simulink model "SensorFaultInj"  (R2013a)
settings: Solver=FixedStepDiscrete  SolverMode=SingleTasking  StartTime=0.0  StopTime=SimLength  FixedStep=SampleTime  RelTol=1e-3
values from neighbouring files (symbols this model uses):
  GlobalSeed = 10    [start_framework07.m]
  SampleTime = 0.01    [start_framework07.m]
  SimLength = 40    [start_framework07.m]
undefined symbols (not defined in the file or in its folder): DiscIntNeverNeededParam
libraries: dspswit3 x48, simulink x32
(part 5 of 9)

== system SensorFaultInj/FIM_Muster1/Parser Modul/schedule once per sample step /schedule_fcn id 2 ==
  In1 : Inport
  Discrete-Time Integrator : DiscreteIntegrator  SampleTime=-1  ICPrevOutput=DiscIntNeverNeededParam  ICPrevScaledInput=DiscIntNeverNeededParam
  Scope1 : Scope  NumInputPorts=2
      settings: YMin=-5~-5  YMax=5~5  SaveName=ScopeData25
  SimLength : Constant  Value=SimLength
  ex_sfun_schedulefcn1 : S-Function  FunctionName=ex_sfun_schedulefcn  EnableBusSupport=off  mask(Legacy Function){SFunctionSpec=single y1 = schedule_fcn(double u1, double u2, single u3, single u4), ShowSpec=on}
      mask prompts: ShowSpec "Display function specification"
      mask help:
      | This block allows you to call the legacy functions specified by the following Legacy Code Tool definition:
      | def.SFunctionName = 'ex_sfun_schedulefcn';
      | def.OutputFcnSpec = 'single y1 = schedule_fcn(double u1, double u2, single u3, single u4)';
      | def.HeaderFiles = {'schedule_fcn.hpp'};
      | def.SourceFiles = {'schedule_fcn.cpp'};
      | def.Options.language = 'C++';
      mask Help: <p>This block was generated automatically by the Legacy Code Tool. For detailed help on this tool, call<a href="matlab:legacy_code('help')"> legacy_code('help')</a>.</p>
      mask Callback ShowSpec:
      | if strcmp(get_param(gcbh, 'ShowSpec'), 'on')
      |   set_param(gcbh, 'MaskDisplay', sprintf('fprintf(''%s'');', get_param(gcbh, 'SFunctionSpec')));
      | else
      |   set_param(gcbh, 'MaskDisplay', sprintf('fprintf(''%s'');', get_param(gcbh, 'FunctionName')));
      | end
      mask Display: fprintf('single y1 = schedule_fcn(double u1, double u2, single u3, single u4)');
  "fault_id " : Constant  Value=2  OutDataTypeStr=single
  one : Constant
  output : Outport  OutputWhenDisabled=reset  InitialOutput=[0]
  wires:
  one/1 -> Discrete-Time Integrator/1
  Discrete-Time Integrator/1 -> ex_sfun_schedulefcn1/2, Scope1/2
  ex_sfun_schedulefcn1/1 -> Scope1/1, output/1  "vcn_schedule"
  SimLength/1 -> ex_sfun_schedulefcn1/1
  "fault_id "/1 -> ex_sfun_schedulefcn1/3
  In1/1 -> ex_sfun_schedulefcn1/4

== system SensorFaultInj/FIM_Muster1/Parser Modul/schedule once per sample step /schedule_fcn id 3 ==
  In1 : Inport
  Discrete-Time Integrator : DiscreteIntegrator  SampleTime=-1  ICPrevOutput=DiscIntNeverNeededParam  ICPrevScaledInput=DiscIntNeverNeededParam
  Scope1 : Scope  NumInputPorts=2
      settings: YMin=-5~-5  YMax=5~5  SaveName=ScopeData25
  SimLength : Constant  Value=SimLength
  ex_sfun_schedulefcn1 : S-Function  FunctionName=ex_sfun_schedulefcn  EnableBusSupport=off  mask(Legacy Function){SFunctionSpec=single y1 = schedule_fcn(double u1, double u2, single u3, single u4), ShowSpec=on}
      mask prompts: ShowSpec "Display function specification"
      mask help:
      | This block allows you to call the legacy functions specified by the following Legacy Code Tool definition:
      | def.SFunctionName = 'ex_sfun_schedulefcn';
      | def.OutputFcnSpec = 'single y1 = schedule_fcn(double u1, double u2, single u3, single u4)';
      | def.HeaderFiles = {'schedule_fcn.hpp'};
      | def.SourceFiles = {'schedule_fcn.cpp'};
      | def.Options.language = 'C++';
      mask Help: <p>This block was generated automatically by the Legacy Code Tool. For detailed help on this tool, call<a href="matlab:legacy_code('help')"> legacy_code('help')</a>.</p>
      mask Callback ShowSpec:
      | if strcmp(get_param(gcbh, 'ShowSpec'), 'on')
      |   set_param(gcbh, 'MaskDisplay', sprintf('fprintf(''%s'');', get_param(gcbh, 'SFunctionSpec')));
      | else
      |   set_param(gcbh, 'MaskDisplay', sprintf('fprintf(''%s'');', get_param(gcbh, 'FunctionName')));
      | end
      mask Display: fprintf('single y1 = schedule_fcn(double u1, double u2, single u3, single u4)');
  "fault_id " : Constant  Value=3  OutDataTypeStr=single
  one : Constant
  output : Outport  OutputWhenDisabled=reset  InitialOutput=[0]
  wires:
  one/1 -> Discrete-Time Integrator/1
  Discrete-Time Integrator/1 -> ex_sfun_schedulefcn1/2, Scope1/2
  ex_sfun_schedulefcn1/1 -> Scope1/1, output/1  "tcn_schedule"
  SimLength/1 -> ex_sfun_schedulefcn1/1
  "fault_id "/1 -> ex_sfun_schedulefcn1/3
  In1/1 -> ex_sfun_schedulefcn1/4

== system SensorFaultInj/FIM_Muster1/Parser Modul/schedule once per sample step /schedule_fcn id 4 ==
  In1 : Inport
  Discrete-Time Integrator : DiscreteIntegrator  SampleTime=-1  ICPrevOutput=DiscIntNeverNeededParam  ICPrevScaledInput=DiscIntNeverNeededParam
  Scope1 : Scope  NumInputPorts=2
      settings: YMin=-5~-5  YMax=5~5  SaveName=ScopeData25
  SimLength : Constant  Value=SimLength
  ex_sfun_schedulefcn1 : S-Function  FunctionName=ex_sfun_schedulefcn  EnableBusSupport=off  mask(Legacy Function){SFunctionSpec=single y1 = schedule_fcn(double u1, double u2, single u3, single u4), ShowSpec=on}
      mask prompts: ShowSpec "Display function specification"
      mask help:
      | This block allows you to call the legacy functions specified by the following Legacy Code Tool definition:
      | def.SFunctionName = 'ex_sfun_schedulefcn';
      | def.OutputFcnSpec = 'single y1 = schedule_fcn(double u1, double u2, single u3, single u4)';
      | def.HeaderFiles = {'schedule_fcn.hpp'};
      | def.SourceFiles = {'schedule_fcn.cpp'};
      | def.Options.language = 'C++';
      mask Help: <p>This block was generated automatically by the Legacy Code Tool. For detailed help on this tool, call<a href="matlab:legacy_code('help')"> legacy_code('help')</a>.</p>
      mask Callback ShowSpec:
      | if strcmp(get_param(gcbh, 'ShowSpec'), 'on')
      |   set_param(gcbh, 'MaskDisplay', sprintf('fprintf(''%s'');', get_param(gcbh, 'SFunctionSpec')));
      | else
      |   set_param(gcbh, 'MaskDisplay', sprintf('fprintf(''%s'');', get_param(gcbh, 'FunctionName')));
      | end
      mask Display: fprintf('single y1 = schedule_fcn(double u1, double u2, single u3, single u4)');
  "fault_id " : Constant  Value=4  OutDataTypeStr=single
  one : Constant
  output : Outport  OutputWhenDisabled=reset  InitialOutput=[0]
  wires:
  one/1 -> Discrete-Time Integrator/1
  Discrete-Time Integrator/1 -> ex_sfun_schedulefcn1/2, Scope1/2
  ex_sfun_schedulefcn1/1 -> Scope1/1, output/1  "nco_schedule"
  SimLength/1 -> ex_sfun_schedulefcn1/1
  "fault_id "/1 -> ex_sfun_schedulefcn1/3
  In1/1 -> ex_sfun_schedulefcn1/4

== system SensorFaultInj/FIM_Muster1/Parser Modul/schedule once per sample step /schedule_fcn id 5 ==
  In1 : Inport
  Discrete-Time Integrator : DiscreteIntegrator  SampleTime=-1  ICPrevOutput=DiscIntNeverNeededParam  ICPrevScaledInput=DiscIntNeverNeededParam
  Scope1 : Scope  NumInputPorts=2
      settings: YMin=-5~-5  YMax=5~5  SaveName=ScopeData25
  SimLength : Constant  Value=SimLength
  ex_sfun_schedulefcn1 : S-Function  FunctionName=ex_sfun_schedulefcn  EnableBusSupport=off  mask(Legacy Function){SFunctionSpec=single y1 = schedule_fcn(double u1, double u2, single u3, single u4), ShowSpec=on}
      mask prompts: ShowSpec "Display function specification"
      mask help:
      | This block allows you to call the legacy functions specified by the following Legacy Code Tool definition:
      | def.SFunctionName = 'ex_sfun_schedulefcn';
      | def.OutputFcnSpec = 'single y1 = schedule_fcn(double u1, double u2, single u3, single u4)';
      | def.HeaderFiles = {'schedule_fcn.hpp'};
      | def.SourceFiles = {'schedule_fcn.cpp'};
      | def.Options.language = 'C++';
      mask Help: <p>This block was generated automatically by the Legacy Code Tool. For detailed help on this tool, call<a href="matlab:legacy_code('help')"> legacy_code('help')</a>.</p>
      mask Callback ShowSpec:
      | if strcmp(get_param(gcbh, 'ShowSpec'), 'on')
      |   set_param(gcbh, 'MaskDisplay', sprintf('fprintf(''%s'');', get_param(gcbh, 'SFunctionSpec')));
      | else
      |   set_param(gcbh, 'MaskDisplay', sprintf('fprintf(''%s'');', get_param(gcbh, 'FunctionName')));
      | end
      mask Display: fprintf('single y1 = schedule_fcn(double u1, double u2, single u3, single u4)');
  "fault_id " : Constant  Value=5  OutDataTypeStr=single
  one : Constant
  output : Outport  OutputWhenDisabled=reset  InitialOutput=[0]
  wires:
  one/1 -> Discrete-Time Integrator/1
  Discrete-Time Integrator/1 -> ex_sfun_schedulefcn1/2, Scope1/2
  ex_sfun_schedulefcn1/1 -> Scope1/1, output/1  "ncn_schedule"
  SimLength/1 -> ex_sfun_schedulefcn1/1
  "fault_id "/1 -> ex_sfun_schedulefcn1/3
  In1/1 -> ex_sfun_schedulefcn1/4

== system SensorFaultInj/FIM_Muster1/Parser Modul/schedule once per sample step /schedule_fcn id 6 ==
  In1 : Inport
  Discrete-Time Integrator : DiscreteIntegrator  SampleTime=-1  ICPrevOutput=DiscIntNeverNeededParam  ICPrevScaledInput=DiscIntNeverNeededParam
  Scope1 : Scope  NumInputPorts=2
      settings: YMin=-5~-5  YMax=5~5  SaveName=ScopeData25
  SimLength : Constant  Value=SimLength
  ex_sfun_schedulefcn1 : S-Function  FunctionName=ex_sfun_schedulefcn  EnableBusSupport=off  mask(Legacy Function){SFunctionSpec=single y1 = schedule_fcn(double u1, double u2, single u3, single u4), ShowSpec=on}
      mask prompts: ShowSpec "Display function specification"
      mask help:
      | This block allows you to call the legacy functions specified by the following Legacy Code Tool definition:
      | def.SFunctionName = 'ex_sfun_schedulefcn';
      | def.OutputFcnSpec = 'single y1 = schedule_fcn(double u1, double u2, single u3, single u4)';
      | def.HeaderFiles = {'schedule_fcn.hpp'};
      | def.SourceFiles = {'schedule_fcn.cpp'};
      | def.Options.language = 'C++';
      mask Help: <p>This block was generated automatically by the Legacy Code Tool. For detailed help on this tool, call<a href="matlab:legacy_code('help')"> legacy_code('help')</a>.</p>
      mask Callback ShowSpec:
      | if strcmp(get_param(gcbh, 'ShowSpec'), 'on')
      |   set_param(gcbh, 'MaskDisplay', sprintf('fprintf(''%s'');', get_param(gcbh, 'SFunctionSpec')));
      | else
      |   set_param(gcbh, 'MaskDisplay', sprintf('fprintf(''%s'');', get_param(gcbh, 'FunctionName')));
      | end
      mask Display: fprintf('single y1 = schedule_fcn(double u1, double u2, single u3, single u4)');
  "fault_id " : Constant  Value=6  OutDataTypeStr=single
  one : Constant
  output : Outport  OutputWhenDisabled=reset  InitialOutput=[0]
  wires:
  one/1 -> Discrete-Time Integrator/1
  Discrete-Time Integrator/1 -> ex_sfun_schedulefcn1/2, Scope1/2
  ex_sfun_schedulefcn1/1 -> Scope1/1, output/1  "out_schedule"
  SimLength/1 -> ex_sfun_schedulefcn1/1
  "fault_id "/1 -> ex_sfun_schedulefcn1/3
  In1/1 -> ex_sfun_schedulefcn1/4

== system SensorFaultInj/FIM_Muster1/Parser Modul/schedule once per sample step /schedule_fcn id 7 ==
  In1 : Inport
  Discrete-Time Integrator : DiscreteIntegrator  SampleTime=-1  ICPrevOutput=DiscIntNeverNeededParam  ICPrevScaledInput=DiscIntNeverNeededParam
  Scope1 : Scope  NumInputPorts=2
      settings: YMin=-5~-5  YMax=5~5  SaveName=ScopeData25
  SimLength : Constant  Value=SimLength
  ex_sfun_schedulefcn1 : S-Function  FunctionName=ex_sfun_schedulefcn  EnableBusSupport=off  mask(Legacy Function){SFunctionSpec=single y1 = schedule_fcn(double u1, double u2, single u3, single u4), ShowSpec=on}
      mask prompts: ShowSpec "Display function specification"
      mask help:
      | This block allows you to call the legacy functions specified by the following Legacy Code Tool definition:
      | def.SFunctionName = 'ex_sfun_schedulefcn';
      | def.OutputFcnSpec = 'single y1 = schedule_fcn(double u1, double u2, single u3, single u4)';
      | def.HeaderFiles = {'schedule_fcn.hpp'};
      | def.SourceFiles = {'schedule_fcn.cpp'};
      | def.Options.language = 'C++';
      mask Help: <p>This block was generated automatically by the Legacy Code Tool. For detailed help on this tool, call<a href="matlab:legacy_code('help')"> legacy_code('help')</a>.</p>
      mask Callback ShowSpec:
      | if strcmp(get_param(gcbh, 'ShowSpec'), 'on')
      |   set_param(gcbh, 'MaskDisplay', sprintf('fprintf(''%s'');', get_param(gcbh, 'SFunctionSpec')));
      | else
      |   set_param(gcbh, 'MaskDisplay', sprintf('fprintf(''%s'');', get_param(gcbh, 'FunctionName')));
      | end
      mask Display: fprintf('single y1 = schedule_fcn(double u1, double u2, single u3, single u4)');
  "fault_id " : Constant  Value=7  OutDataTypeStr=single
  one : Constant
  output : Outport  OutputWhenDisabled=reset  InitialOutput=[0]
  wires:
  one/1 -> Discrete-Time Integrator/1
  Discrete-Time Integrator/1 -> ex_sfun_schedulefcn1/2, Scope1/2
  ex_sfun_schedulefcn1/1 -> Scope1/1, output/1  "spi_schedule"
  SimLength/1 -> ex_sfun_schedulefcn1/1
  "fault_id "/1 -> ex_sfun_schedulefcn1/3
  In1/1 -> ex_sfun_schedulefcn1/4

== system SensorFaultInj/FIM_Muster1/Parser Modul/schedule once per sample step /schedule_fcn id 8 ==
  In1 : Inport
  Discrete-Time Integrator : DiscreteIntegrator  SampleTime=-1  ICPrevOutput=DiscIntNeverNeededParam  ICPrevScaledInput=DiscIntNeverNeededParam
  Scope1 : Scope  NumInputPorts=2
      settings: YMin=-5~-5  YMax=5~5  SaveName=ScopeData25
  SimLength : Constant  Value=SimLength
  ex_sfun_schedulefcn1 : S-Function  FunctionName=ex_sfun_schedulefcn  EnableBusSupport=off  mask(Legacy Function){SFunctionSpec=single y1 = schedule_fcn(double u1, double u2, single u3, single u4), ShowSpec=on}
      mask prompts: ShowSpec "Display function specification"
      mask help:
      | This block allows you to call the legacy functions specified by the following Legacy Code Tool definition:
      | def.SFunctionName = 'ex_sfun_schedulefcn';
      | def.OutputFcnSpec = 'single y1 = schedule_fcn(double u1, double u2, single u3, single u4)';
      | def.HeaderFiles = {'schedule_fcn.hpp'};
      | def.SourceFiles = {'schedule_fcn.cpp'};
      | def.Options.language = 'C++';
      mask Help: <p>This block was generated automatically by the Legacy Code Tool. For detailed help on this tool, call<a href="matlab:legacy_code('help')"> legacy_code('help')</a>.</p>
      mask Callback ShowSpec:
      | if strcmp(get_param(gcbh, 'ShowSpec'), 'on')
      |   set_param(gcbh, 'MaskDisplay', sprintf('fprintf(''%s'');', get_param(gcbh, 'SFunctionSpec')));
      | else
      |   set_param(gcbh, 'MaskDisplay', sprintf('fprintf(''%s'');', get_param(gcbh, 'FunctionName')));
      | end
      mask Display: fprintf('single y1 = schedule_fcn(double u1, double u2, single u3, single u4)');
  "fault_id " : Constant  Value=8  OutDataTypeStr=single
  one : Constant
  output : Outport  OutputWhenDisabled=reset  InitialOutput=[0]
  wires:
  one/1 -> Discrete-Time Integrator/1
  Discrete-Time Integrator/1 -> ex_sfun_schedulefcn1/2, Scope1/2
  ex_sfun_schedulefcn1/1 -> Scope1/1, output/1  "stz_schedule"
  SimLength/1 -> ex_sfun_schedulefcn1/1
  "fault_id "/1 -> ex_sfun_schedulefcn1/3
  In1/1 -> ex_sfun_schedulefcn1/4

== system SensorFaultInj/FIM_Muster1/Parser Modul/schedule once per sample step /schedule_fcn id 9 ==
  In1 : Inport
  Discrete-Time Integrator : DiscreteIntegrator  SampleTime=-1  ICPrevOutput=DiscIntNeverNeededParam  ICPrevScaledInput=DiscIntNeverNeededParam
  Scope1 : Scope  NumInputPorts=2
      settings: YMin=-5~-5  YMax=5~5  SaveName=ScopeData25
  SimLength : Constant  Value=SimLength
  ex_sfun_schedulefcn1 : S-Function  FunctionName=ex_sfun_schedulefcn  EnableBusSupport=off  mask(Legacy Function){SFunctionSpec=single y1 = schedule_fcn(double u1, double u2, single u3, single u4), ShowSpec=on}
      mask prompts: ShowSpec "Display function specification"
      mask help:
      | This block allows you to call the legacy functions specified by the following Legacy Code Tool definition:
      | def.SFunctionName = 'ex_sfun_schedulefcn';
      | def.OutputFcnSpec = 'single y1 = schedule_fcn(double u1, double u2, single u3, single u4)';
      | def.HeaderFiles = {'schedule_fcn.hpp'};
      | def.SourceFiles = {'schedule_fcn.cpp'};
      | def.Options.language = 'C++';
      mask Help: <p>This block was generated automatically by the Legacy Code Tool. For detailed help on this tool, call<a href="matlab:legacy_code('help')"> legacy_code('help')</a>.</p>
      mask Callback ShowSpec:
      | if strcmp(get_param(gcbh, 'ShowSpec'), 'on')
      |   set_param(gcbh, 'MaskDisplay', sprintf('fprintf(''%s'');', get_param(gcbh, 'SFunctionSpec')));
      | else
      |   set_param(gcbh, 'MaskDisplay', sprintf('fprintf(''%s'');', get_param(gcbh, 'FunctionName')));
      | end
      mask Display: fprintf('single y1 = schedule_fcn(double u1, double u2, single u3, single u4)');
  "fault_id " : Constant  Value=9  OutDataTypeStr=single
  one : Constant
  output : Outport  OutputWhenDisabled=reset  InitialOutput=[0]
  wires:
  one/1 -> Discrete-Time Integrator/1
  Discrete-Time Integrator/1 -> ex_sfun_schedulefcn1/2, Scope1/2
  ex_sfun_schedulefcn1/1 -> Scope1/1, output/1  "stx_schedule"
  SimLength/1 -> ex_sfun_schedulefcn1/1
  "fault_id "/1 -> ex_sfun_schedulefcn1/3
  In1/1 -> ex_sfun_schedulefcn1/4

== system SensorFaultInj/FIM_Muster2/Fault Injection Modul/AFI - additive faults injection/non correated noise ==
  "konf " : Inport
  flank : Inport  Port=2
  xml_id : Inport  Port=3
  Enable : EnablePort
  Product : Product
  Scope : Scope
      settings: SaveName=ScopeData4
  Switch : Switch  Threshold=1
  pdf_parser : Subsystem
  zero : Constant  Value=0
  output : Outport  OutputWhenDisabled=reset  InitialOutput=[0]
  wires:
  zero/1 -> Switch/3
  Switch/1 -> output/1
  flank/1 -> Switch/2
  pdf_parser/1(distr value) -> Product/1
  Product/1 -> Switch/1, Scope/1
  "konf "/1 -> Product/2
  xml_id/1 -> pdf_parser/1(xml id)

== system SensorFaultInj/FIM_Muster2/Fault Injection Modul/AFI - additive faults injection/non correlated offset ==
  konf : Inport
  Enable : EnablePort
  output : Outport  OutputWhenDisabled=reset  InitialOutput=[0]
  wires:
  konf/1 -> output/1

== system SensorFaultInj/FIM_Muster2/Fault Injection Modul/AFI - additive faults injection/outlier ==
  konf : Inport
  flank : Inport  Port=2
  Enable : EnablePort
  Add : Sum
  Bus Selector : BusSelector  OutputSignals=out_amplitude,out_neg
  Interpreted MATLAB Function : MATLABFcn  MATLABFcn=rand
  Interpreted MATLAB Function1 : MATLABFcn  Commented=on
  Product : Product
  Product1 : Product
  Product2 : Product
  Switch1 : Switch  Threshold=1
  Switch2 : Switch  Threshold=1
  const : Constant
  const1 : Constant  Value=-0.5
  const2 : Constant  Value=0
  const3 : Constant  Value=2
  output : Outport  OutputWhenDisabled=reset  InitialOutput=[0]
  wires:
  const/1 -> Interpreted MATLAB Function/1
  Interpreted MATLAB Function/1 -> Add/1, Product/2
  const1/1 -> Add/2
  Add/1 -> Product1/1
  Product/1 -> Switch1/3
  Switch1/1 -> Switch2/1
  Bus Selector/2 -> Switch1/2  "<out_neg>"
  Bus Selector/1 -> Product/1, Product1/2  "<out_amplitude>"
  konf/1 -> Bus Selector/1
  Switch2/1 -> output/1
  flank/1 -> Switch2/2
  const2/1 -> Switch2/3
  const3/1 -> Product2/1
  Product1/1 -> Product2/2
  Product2/1 -> Switch1/1

== system SensorFaultInj/FIM_Muster2/Fault Injection Modul/AFI - additive faults injection/spike ==
  konf : Inport
  flank : Inport  Port=2
  xml_id : Inport  Port=3
  Enable : EnablePort  StatesWhenEnabling=reset
  Bus Selector : BusSelector  OutputSignals=spi_length,spi_factor
  Constant : Constant
  Constant1 : Constant  Value=0
  Constant2 : Constant  Value=7  OutDataTypeStr=single
  Discrete-Time Integrator : DiscreteIntegrator  gainval=1  ExternalReset=falling  SampleTime=SampleTime  ICPrevOutput=DiscIntNeverNeededParam  ICPrevScaledInput=DiscIntNeverNeededParam
  Product : Product
  Switch : Switch  Threshold=1
  ex_sfun_spikefcn : S-Function  FunctionName=ex_sfun_spikefcn  EnableBusSupport=off  mask(Legacy Function){SFunctionSpec=double y1 = spike_fcn(single u1, single u2, double u3, double u4), ShowSpec=on}
      mask prompts: ShowSpec "Display function specification"
      mask help:
      | This block allows you to call the legacy functions specified by the following Legacy Code Tool definition:
      | def.SFunctionName = 'ex_sfun_spikefcn';
      | def.OutputFcnSpec = 'double y1 = spike_fcn(single u1, single u2, double u3, double u4)';
      | def.HeaderFiles = {'spike_fcn.hpp'};
      | def.SourceFiles = {'spike_fcn.cpp'};
      | def.Options.language = 'C++';
      mask Help: <p>This block was generated automatically by the Legacy Code Tool. For detailed help on this tool, call<a href="matlab:legacy_code('help')"> legacy_code('help')</a>.</p>
      mask Callback ShowSpec:
      | if strcmp(get_param(gcbh, 'ShowSpec'), 'on')
      |   set_param(gcbh, 'MaskDisplay', sprintf('fprintf(''%s'');', get_param(gcbh, 'SFunctionSpec')));
      | else
      |   set_param(gcbh, 'MaskDisplay', sprintf('fprintf(''%s'');', get_param(gcbh, 'FunctionName')));
      | end
      mask Display: fprintf('double y1 = spike_fcn(single u1, single u2, double u3, double u4)');
  output : Outport  OutputWhenDisabled=reset  InitialOutput=[0]
  wires:
  Constant1/1 -> Switch/3
  Switch/1 -> Discrete-Time Integrator/1
  flank/1 -> Discrete-Time Integrator/2, Switch/2
  Constant/1 -> Switch/1
  Discrete-Time Integrator/1 -> ex_sfun_spikefcn/4
  xml_id/1 -> ex_sfun_spikefcn/2
  Constant2/1 -> ex_sfun_spikefcn/1
  Product/1 -> output/1
  konf/1 -> Bus Selector/1
  Bus Selector/1 -> ex_sfun_spikefcn/3  "<spi_length>"
  ex_sfun_spikefcn/1 -> Product/2
  Bus Selector/2 -> Product/1  "<spi_factor>"

== system SensorFaultInj/FIM_Muster2/Fault Injection Modul/AFI - additive faults injection/stuck at x generation ==
  input : Inport
  konf : Inport  Port=2
  flank : Inport  Port=3
  enable : Inport  Port=4
  Bus Selector : BusSelector  OutputSignals=stx_min,stx_max
  Switch1 : Switch  Threshold=1
  Switch2 : Switch  Threshold=1
  Triggered Subsystem1 : Subsystem  TreatAsAtomicUnit=on
  output : Outport
  wires:
  konf/1 -> Bus Selector/1
  input/1 -> Switch2/3, Switch1/3, Triggered Subsystem1/1("In1 ")
  flank/1 -> Switch1/2, Triggered Subsystem1/Trigger
  Triggered Subsystem1/1(Out1) -> Switch1/1
  enable/1 -> Switch2/2
  Switch1/1 -> Switch2/1
  Switch2/1 -> output/1

== system SensorFaultInj/FIM_Muster2/Fault Injection Modul/AFI - additive faults injection/stuck at x generation1 ==
  input : Inport
  konf : Inport  Port=2
  flank : Inport  Port=3
  enable : Inport  Port=4
  Bus Selector : BusSelector  OutputSignals=stx_min,stx_max
  Switch1 : Switch  Threshold=1
  Switch2 : Switch  Threshold=1
  Triggered Subsystem : Subsystem  TreatAsAtomicUnit=on
  output : Outport
  wires:
  konf/1 -> Bus Selector/1
  Bus Selector/2 -> Triggered Subsystem/2(bottom border)  "<stx_max>"
  Bus Selector/1 -> Triggered Subsystem/1(top border)  "<stx_min>"
  input/1 -> Switch2/3, Switch1/3
  flank/1 -> Triggered Subsystem/Trigger, Switch1/2
  Triggered Subsystem/1(Out1) -> Switch1/1
  enable/1 -> Switch2/2
  Switch1/1 -> Switch2/1
  Switch2/1 -> output/1

== system SensorFaultInj/FIM_Muster2/Fault Injection Modul/AFI - additive faults injection/stuck at zero generation ==
  input : Inport
  flank : Inport  Port=2
  enable : Inport  Port=3
  Constant : Constant  Value=0
  Switch : Switch  Threshold=1
  Switch1 : Switch  Threshold=1
  output : Outport
  wires:
  Switch/1 -> Switch1/1
  Switch1/1 -> output/1
  enable/1 -> Switch1/2
  input/1 -> Switch/3, Switch1/3
  Constant/1 -> Switch/1
  flank/1 -> Switch/2

== system SensorFaultInj/FIM_Muster2/Fault Injection Modul/FFI - functional fault injection/const delay  ==
  input : Inport
  konf : Inport  Port=2
  enable : Inport  Port=3
  Switch : Switch  Criteria=u2 ~= 0
  Variable Time Delay : VariableTransportDelay  MaximumDelay=10
  Zero-Order Hold : ZeroOrderHold  SampleTime=SampleTime
  output1 : Outport  OutputWhenDisabled=reset  InitialOutput=[0]
  delay : Outport  Port=2  OutputWhenDisabled=reset  InitialOutput=[0]
  wires:
  input/1 -> Switch/3, Variable Time Delay/1
  Switch/1 -> output1/1
  enable/1 -> Switch/2
  konf/1 -> delay/1, Variable Time Delay/2
  Variable Time Delay/1 -> Zero-Order Hold/1
  Zero-Order Hold/1 -> Switch/1

== system SensorFaultInj/FIM_Muster2/Fault Injection Modul/FFI - functional fault injection/saturation ==
  input : Inport
  "konf " : Inport  Port=2
  enable : Inport  Port=3
  Demux1 : Demux  Outputs=2
  Divide : Product  Inputs=*/
  Divide1 : Product  Inputs=*/
  Switch : Switch  Criteria=u2 ~= 0
  Switch1 : Switch  Threshold=1
  Switch2 : Switch  Threshold=1
  output : Outport  OutputWhenDisabled=reset  InitialOutput=[0]
  wires:
  input/1 -> Switch/3, Switch1/3, Divide/1
  Divide/1 -> Switch1/2
  Switch1/1 -> Divide1/1, Switch2/3
  Divide1/1 -> Switch2/2
  Switch2/1 -> Switch/1
  Demux1/1 -> Switch1/1, Divide/2
  Demux1/2 -> Switch2/1, Divide1/2
  "konf "/1 -> Demux1/1
  Switch/1 -> output/1
  enable/1 -> Switch/2

== system SensorFaultInj/FIM_Muster2/Fault Injection Modul/FFI - functional fault injection/time correlated delay  ==
  input : Inport
  konf : Inport  Port=2
  enable : Inport  Port=3
  xml id : Inport  Port=4
  Gain : Gain  Gain=-1
  Product : Product
  Product1 : Product
  Switch : Switch  Criteria=u2 ~= 0
  Switch1 : Switch  Criteria=u2 > Threshold
  Variable Time Delay : VariableTransportDelay  MaximumDelay=10  ZeroDelay=on
  Zero-Order Hold : ZeroOrderHold  SampleTime=SampleTime
  amplitude : Constant
  const : Constant  Value=0
  expr_parser : Subsystem
  output1 : Outport  OutputWhenDisabled=reset  InitialOutput=[0]
  delay : Outport  Port=2  OutputWhenDisabled=reset  InitialOutput=[0]
  wires:
  input/1 -> Switch/3, Variable Time Delay/1
  Switch/1 -> output1/1
  enable/1 -> Switch/2
  konf/1 -> Product/2
  Switch1/1 -> delay/1, Variable Time Delay/2
  Product1/1 -> Product/1
  amplitude/1 -> Product1/1
  expr_parser/1(corelation value) -> Product1/2
  xml id/1 -> expr_parser/1(xml id)
  Variable Time Delay/1 -> Zero-Order Hold/1
  Zero-Order Hold/1 -> Switch/1
  Gain/1 -> Switch1/2
  const/1 -> Switch1/1
  Product/1 -> Switch1/3, Gain/1

== system SensorFaultInj/FIM_Muster2/Fault Injection Modul/MFI - multiplicative fault injection/time correlated noise ==
  konf : Inport
  flank : Inport  Port=2
  xml id : Inport  Port=3
  Enable : EnablePort
  Product2 : Product  Inputs=3
  Scope : Scope
      settings: SaveName=ScopeData21
  Switch1 : Switch  Threshold=1
  expr_parser1 : Subsystem
  pdf_parser : Subsystem
  zero : Constant  Value=0
  output : Outport  OutputWhenDisabled=reset  InitialOutput=[0]
  wires:
  flank/1 -> Switch1/2
  Switch1/1 -> output/1
  zero/1 -> Switch1/3
  expr_parser1/1(corelation value) -> Product2/1
  xml id/1 -> pdf_parser/1(xml id), expr_parser1/1(xml id)
  konf/1 -> Product2/3
  pdf_parser/1(distr value) -> Product2/2
  Product2/1 -> Switch1/1, Scope/1

== system SensorFaultInj/FIM_Muster2/Fault Injection Modul/MFI - multiplicative fault injection/time correlated offset ==
  konf : Inport
  xml id : Inport  Port=2
  Enable : EnablePort
  Product : Product
  Scope : Scope  NumInputPorts=2
      settings: TimeRange=10  YMin=-5~-5  YMax=5~5  SaveName=ScopeData22
  expr_parser : Subsystem
  output : Outport  OutputWhenDisabled=reset  InitialOutput=[0]
  wires:
  Product/1 -> Scope/1, output/1
  expr_parser/1(corelation value) -> Product/2, Scope/2
  konf/1 -> Product/1
  xml id/1 -> expr_parser/1(xml id)

== system SensorFaultInj/FIM_Muster2/Fault Injection Modul/MFI - multiplicative fault injection/value correlated noise ==
  input : Inport
  konf : Inport  Port=2
  flank : Inport  Port=3
  xml_id : Inport  Port=4
  Enable : EnablePort
  Product1 : Product  RndMeth=Zero
  Product2 : Product  RndMeth=Zero
  Switch : Switch  Threshold=1
  pdf_parser : Subsystem
  zero : Constant  Value=0
  output : Outport  OutputWhenDisabled=reset  InitialOutput=[0]
  wires:
  zero/1 -> Switch/3
  Switch/1 -> output/1
  input/1 -> Product2/1
  pdf_parser/1(distr value) -> Product1/2
  Product2/1 -> Product1/1
  Product1/1 -> Switch/1
  flank/1 -> Switch/2
  xml_id/1 -> pdf_parser/1(xml id)
  konf/1 -> Product2/2

== system SensorFaultInj/FIM_Muster2/Fault Injection Modul/MFI - multiplicative fault injection/value correlated offset ==
  input : Inport
  konf : Inport  Port=2
  Enable : EnablePort
  Product : Product  RndMeth=Zero
  Subtract : Sum  Inputs=+-
  output : Outport  OutputWhenDisabled=reset  InitialOutput=[0]
  wires:
  input/1 -> Subtract/1, Product/1
  konf/1 -> Product/2
  Product/1 -> Subtract/2
  Subtract/1 -> output/1

== system SensorFaultInj/FIM_Muster2/Parser Modul/occurence parser /Enabled Subsystem ==
  In1 : Inport
  Enable : EnablePort
  Bus Creator : BusCreator  Inputs=7
  occurnce parser fault id 2 : Subsystem
  occurnce parser fault id 3 : Subsystem
  occurnce parser fault id 5 : Subsystem
  occurnce parser fault id 6 : Subsystem
  occurnce parser fault id 7 : Subsystem
  occurnce parser fault id 8 : Subsystem
  occurnce parser fault id 9 : Subsystem
  Out1 : Outport
  wires:
  occurnce parser fault id 8/1(Out1) -> Bus Creator/6
  occurnce parser fault id 5/1(Out1) -> Bus Creator/3
  occurnce parser fault id 7/1(Out1) -> Bus Creator/5
  occurnce parser fault id 6/1(Out1) -> Bus Creator/4
  occurnce parser fault id 2/1(Out1) -> Bus Creator/1
  occurnce parser fault id 3/1(Out1) -> Bus Creator/2
  occurnce parser fault id 9/1(Out1) -> Bus Creator/7
  Bus Creator/1 -> Out1/1  "occurrence_bus"
  In1/1 -> occurnce parser fault id 3/1(In1), occurnce parser fault id 5/1(In1), occurnce parser fault id 6/1(In1), occurnce parser fault id 7/1(In1), occurnce parser fault id 8/1(In1), occurnce parser fault id 9/1(In1), occurnce parser fault id 2/1(In1)

== system SensorFaultInj/FIM_Muster2/Parser Modul/parameter parser/Enabled Subsystem ==
  In1 : Inport
  Enable : EnablePort
  Bus Creator : BusCreator  Inputs=13
  param_fcn id 0 : Subsystem
  param_fcn id 1 : Subsystem
  param_fcn id 10 : Subsystem
  param_fcn id 11 : Subsystem
  param_fcn id 12 : Subsystem
  param_fcn id 2 : Subsystem
  param_fcn id 3 : Subsystem
  param_fcn id 4 : Subsystem
  param_fcn id 5 : Subsystem
  param_fcn id 6 : Subsystem
  param_fcn id 7 : Subsystem
  param_fcn id 8 : Subsystem
  param_fcn id 9 : Subsystem
  Out1 : Outport  LockScale=on
  wires:
  Bus Creator/1 -> Out1/1  "parameter_bus"
  In1/1 -> param_fcn id 1/1(In1), param_fcn id 3/1(In1), param_fcn id 5/1(In1), param_fcn id 6/1(In1), param_fcn id 7/1(In1), param_fcn id 8/1(In1), param_fcn id 9/1(In1), param_fcn id 10/1(In1), param_fcn id 12/1(In1), param_fcn id 11/1(In1), param_fcn id 4/1(In1), param_fcn id 2/1(In1), param_fcn id 0/1(In1)
  param_fcn id 8/1(Out1) -> Bus Creator/9
  param_fcn id 4/1(Out1) -> Bus Creator/5
  param_fcn id 6/1(Out1) -> Bus Creator/7
  param_fcn id 2/1(Out1) -> Bus Creator/3
  param_fcn id 1/1(Out1) -> Bus Creator/2
  param_fcn id 3/1(Out1) -> Bus Creator/4
  param_fcn id 7/1(Out1) -> Bus Creator/8
  param_fcn id 0/1(Out1) -> Bus Creator/1
  param_fcn id 5/1(Out1) -> Bus Creator/6
  param_fcn id 11/1(Out1) -> Bus Creator/12
  param_fcn id 12/1(Out1) -> Bus Creator/13
  param_fcn id 9/1(Out1) -> Bus Creator/10
  param_fcn id 10/1(Out1) -> Bus Creator/11

== system SensorFaultInj/FIM_Muster2/Parser Modul/schedule once per sample step /schedule_fcn id 0 ==
  In1 : Inport
  Discrete-Time Integrator : DiscreteIntegrator  SampleTime=-1  ICPrevOutput=DiscIntNeverNeededParam  ICPrevScaledInput=DiscIntNeverNeededParam
  Scope1 : Scope  NumInputPorts=2
      settings: YMin=-5~-5  YMax=5~5  SaveName=ScopeData25
  SimLength : Constant  Value=SimLength
  ex_sfun_schedulefcn1 : S-Function  FunctionName=ex_sfun_schedulefcn  EnableBusSupport=off  mask(Legacy Function){SFunctionSpec=single y1 = schedule_fcn(double u1, double u2, single u3, single u4), ShowSpec=on}
      mask prompts: ShowSpec "Display function specification"
      mask help:
      | This block allows you to call the legacy functions specified by the following Legacy Code Tool definition:
      | def.SFunctionName = 'ex_sfun_schedulefcn';
      | def.OutputFcnSpec = 'single y1 = schedule_fcn(double u1, double u2, single u3, single u4)';
      | def.HeaderFiles = {'schedule_fcn.hpp'};
      | def.SourceFiles = {'schedule_fcn.cpp'};
      | def.Options.language = 'C++';
      mask Help: <p>This block was generated automatically by the Legacy Code Tool. For detailed help on this tool, call<a href="matlab:legacy_code('help')"> legacy_code('help')</a>.</p>
      mask Callback ShowSpec:
      | if strcmp(get_param(gcbh, 'ShowSpec'), 'on')
      |   set_param(gcbh, 'MaskDisplay', sprintf('fprintf(''%s'');', get_param(gcbh, 'SFunctionSpec')));
      | else
      |   set_param(gcbh, 'MaskDisplay', sprintf('fprintf(''%s'');', get_param(gcbh, 'FunctionName')));
      | end
      mask Display: fprintf('single y1 = schedule_fcn(double u1, double u2, single u3, single u4)');
  "fault_id " : Constant  Value=0  OutDataTypeStr=single
  one : Constant
  output : Outport  OutputWhenDisabled=reset  InitialOutput=[0]
  wires:
  one/1 -> Discrete-Time Integrator/1
  Discrete-Time Integrator/1 -> ex_sfun_schedulefcn1/2, Scope1/2
  ex_sfun_schedulefcn1/1 -> Scope1/1, output/1  "vco_schedule"
  SimLength/1 -> ex_sfun_schedulefcn1/1
  "fault_id "/1 -> ex_sfun_schedulefcn1/3
  In1/1 -> ex_sfun_schedulefcn1/4

== system SensorFaultInj/FIM_Muster2/Parser Modul/schedule once per sample step /schedule_fcn id 1 ==
  In1 : Inport
  Discrete-Time Integrator : DiscreteIntegrator  SampleTime=-1  ICPrevOutput=DiscIntNeverNeededParam  ICPrevScaledInput=DiscIntNeverNeededParam
  Scope1 : Scope  NumInputPorts=2
      settings: YMin=-5~-5  YMax=5~5  SaveName=ScopeData25
  SimLength : Constant  Value=SimLength
  ex_sfun_schedulefcn1 : S-Function  FunctionName=ex_sfun_schedulefcn  EnableBusSupport=off  mask(Legacy Function){SFunctionSpec=single y1 = schedule_fcn(double u1, double u2, single u3, single u4), ShowSpec=on}
      mask prompts: ShowSpec "Display function specification"
      mask help:
      | This block allows you to call the legacy functions specified by the following Legacy Code Tool definition:
      | def.SFunctionName = 'ex_sfun_schedulefcn';
      | def.OutputFcnSpec = 'single y1 = schedule_fcn(double u1, double u2, single u3, single u4)';
      | def.HeaderFiles = {'schedule_fcn.hpp'};
      | def.SourceFiles = {'schedule_fcn.cpp'};
      | def.Options.language = 'C++';
      mask Help: <p>This block was generated automatically by the Legacy Code Tool. For detailed help on this tool, call<a href="matlab:legacy_code('help')"> legacy_code('help')</a>.</p>
      mask Callback ShowSpec:
      | if strcmp(get_param(gcbh, 'ShowSpec'), 'on')
      |   set_param(gcbh, 'MaskDisplay', sprintf('fprintf(''%s'');', get_param(gcbh, 'SFunctionSpec')));
      | else
      |   set_param(gcbh, 'MaskDisplay', sprintf('fprintf(''%s'');', get_param(gcbh, 'FunctionName')));
      | end
      mask Display: fprintf('single y1 = schedule_fcn(double u1, double u2, single u3, single u4)');
  "fault_id " : Constant  OutDataTypeStr=single
  one : Constant
  output : Outport  OutputWhenDisabled=reset  InitialOutput=[0]
  wires:
  one/1 -> Discrete-Time Integrator/1
  ex_sfun_schedulefcn1/1 -> Scope1/1, output/1  "tco_schedule"
  Discrete-Time Integrator/1 -> ex_sfun_schedulefcn1/2, Scope1/2
  SimLength/1 -> ex_sfun_schedulefcn1/1
  "fault_id "/1 -> ex_sfun_schedulefcn1/3
  In1/1 -> ex_sfun_schedulefcn1/4

== system SensorFaultInj/FIM_Muster2/Parser Modul/schedule once per sample step /schedule_fcn id 10 ==
  In1 : Inport
  Discrete-Time Integrator : DiscreteIntegrator  SampleTime=-1  ICPrevOutput=DiscIntNeverNeededParam  ICPrevScaledInput=DiscIntNeverNeededParam
  Scope1 : Scope  NumInputPorts=2
      settings: YMin=-5~-5  YMax=5~5  SaveName=ScopeData25
  SimLength : Constant  Value=SimLength
  ex_sfun_schedulefcn1 : S-Function  FunctionName=ex_sfun_schedulefcn  EnableBusSupport=off  mask(Legacy Function){SFunctionSpec=single y1 = schedule_fcn(double u1, double u2, single u3, single u4), ShowSpec=on}
      mask prompts: ShowSpec "Display function specification"
      mask help:
      | This block allows you to call the legacy functions specified by the following Legacy Code Tool definition:
      | def.SFunctionName = 'ex_sfun_schedulefcn';
      | def.OutputFcnSpec = 'single y1 = schedule_fcn(double u1, double u2, single u3, single u4)';
      | def.HeaderFiles = {'schedule_fcn.hpp'};
      | def.SourceFiles = {'schedule_fcn.cpp'};
      | def.Options.language = 'C++';
      mask Help: <p>This block was generated automatically by the Legacy Code Tool. For detailed help on this tool, call<a href="matlab:legacy_code('help')"> legacy_code('help')</a>.</p>
      mask Callback ShowSpec:
      | if strcmp(get_param(gcbh, 'ShowSpec'), 'on')
      |   set_param(gcbh, 'MaskDisplay', sprintf('fprintf(''%s'');', get_param(gcbh, 'SFunctionSpec')));
      | else
      |   set_param(gcbh, 'MaskDisplay', sprintf('fprintf(''%s'');', get_param(gcbh, 'FunctionName')));
      | end
      mask Display: fprintf('single y1 = schedule_fcn(double u1, double u2, single u3, single u4)');
  "fault_id " : Constant  Value=10  OutDataTypeStr=single
  one : Constant
  output : Outport  OutputWhenDisabled=reset  InitialOutput=[0]
  wires:
  one/1 -> Discrete-Time Integrator/1
  Discrete-Time Integrator/1 -> ex_sfun_schedulefcn1/2, Scope1/2
  ex_sfun_schedulefcn1/1 -> Scope1/1, output/1  "sat_schedule"
  SimLength/1 -> ex_sfun_schedulefcn1/1
  "fault_id "/1 -> ex_sfun_schedulefcn1/3
  In1/1 -> ex_sfun_schedulefcn1/4

== system SensorFaultInj/FIM_Muster2/Parser Modul/schedule once per sample step /schedule_fcn id 11 ==
  In1 : Inport
  Discrete-Time Integrator : DiscreteIntegrator  SampleTime=-1  ICPrevOutput=DiscIntNeverNeededParam  ICPrevScaledInput=DiscIntNeverNeededParam
  Scope1 : Scope  NumInputPorts=2
      settings: YMin=-5~-5  YMax=5~5  SaveName=ScopeData25
  SimLength : Constant  Value=SimLength
  ex_sfun_schedulefcn1 : S-Function  FunctionName=ex_sfun_schedulefcn  EnableBusSupport=off  mask(Legacy Function){SFunctionSpec=single y1 = schedule_fcn(double u1, double u2, single u3, single u4), ShowSpec=on}
      mask prompts: ShowSpec "Display function specification"
      mask help:
      | This block allows you to call the legacy functions specified by the following Legacy Code Tool definition:
      | def.SFunctionName = 'ex_sfun_schedulefcn';
      | def.OutputFcnSpec = 'single y1 = schedule_fcn(double u1, double u2, single u3, single u4)';
      | def.HeaderFiles = {'schedule_fcn.hpp'};
      | def.SourceFiles = {'schedule_fcn.cpp'};
      | def.Options.language = 'C++';
      mask Help: <p>This block was generated automatically by the Legacy Code Tool. For detailed help on this tool, call<a href="matlab:legacy_code('help')"> legacy_code('help')</a>.</p>
      mask Callback ShowSpec:
      | if strcmp(get_param(gcbh, 'ShowSpec'), 'on')
      |   set_param(gcbh, 'MaskDisplay', sprintf('fprintf(''%s'');', get_param(gcbh, 'SFunctionSpec')));
      | else
      |   set_param(gcbh, 'MaskDisplay', sprintf('fprintf(''%s'');', get_param(gcbh, 'FunctionName')));
      | end
      mask Display: fprintf('single y1 = schedule_fcn(double u1, double u2, single u3, single u4)');
  "fault_id " : Constant  Value=11  OutDataTypeStr=single
  one : Constant
  output : Outport  OutputWhenDisabled=reset  InitialOutput=[0]
  wires:
  one/1 -> Discrete-Time Integrator/1
  Discrete-Time Integrator/1 -> ex_sfun_schedulefcn1/2, Scope1/2
  ex_sfun_schedulefcn1/1 -> Scope1/1, output/1  "ncd_schedule"
  SimLength/1 -> ex_sfun_schedulefcn1/1
  "fault_id "/1 -> ex_sfun_schedulefcn1/3
  In1/1 -> ex_sfun_schedulefcn1/4

== system SensorFaultInj/FIM_Muster2/Parser Modul/schedule once per sample step /schedule_fcn id 12 ==
  In1 : Inport
  Discrete-Time Integrator : DiscreteIntegrator  SampleTime=-1  ICPrevOutput=DiscIntNeverNeededParam  ICPrevScaledInput=DiscIntNeverNeededParam
  Scope1 : Scope  NumInputPorts=2
      settings: YMin=-5~-5  YMax=5~5  SaveName=ScopeData25
  SimLength : Constant  Value=SimLength
  ex_sfun_schedulefcn1 : S-Function  FunctionName=ex_sfun_schedulefcn  EnableBusSupport=off  mask(Legacy Function){SFunctionSpec=single y1 = schedule_fcn(double u1, double u2, single u3, single u4), ShowSpec=on}
      mask prompts: ShowSpec "Display function specification"
      mask help:
      | This block allows you to call the legacy functions specified by the following Legacy Code Tool definition:
      | def.SFunctionName = 'ex_sfun_schedulefcn';
      | def.OutputFcnSpec = 'single y1 = schedule_fcn(double u1, double u2, single u3, single u4)';
      | def.HeaderFiles = {'schedule_fcn.hpp'};
      | def.SourceFiles = {'schedule_fcn.cpp'};
      | def.Options.language = 'C++';
      mask Help: <p>This block was generated automatically by the Legacy Code Tool. For detailed help on this tool, call<a href="matlab:legacy_code('help')"> legacy_code('help')</a>.</p>
      mask Callback ShowSpec:
      | if strcmp(get_param(gcbh, 'ShowSpec'), 'on')
      |   set_param(gcbh, 'MaskDisplay', sprintf('fprintf(''%s'');', get_param(gcbh, 'SFunctionSpec')));
      | else
      |   set_param(gcbh, 'MaskDisplay', sprintf('fprintf(''%s'');', get_param(gcbh, 'FunctionName')));
      | end
      mask Display: fprintf('single y1 = schedule_fcn(double u1, double u2, single u3, single u4)');
  "fault_id " : Constant  Value=12  OutDataTypeStr=single
  one : Constant
  output : Outport  OutputWhenDisabled=reset  InitialOutput=[0]
  wires:
  one/1 -> Discrete-Time Integrator/1
  Discrete-Time Integrator/1 -> ex_sfun_schedulefcn1/2, Scope1/2
  ex_sfun_schedulefcn1/1 -> Scope1/1, output/1  "tcd_schedule"
  SimLength/1 -> ex_sfun_schedulefcn1/1
  "fault_id "/1 -> ex_sfun_schedulefcn1/3
  In1/1 -> ex_sfun_schedulefcn1/4

== system SensorFaultInj/FIM_Muster2/Parser Modul/schedule once per sample step /schedule_fcn id 2 ==
  In1 : Inport
  Discrete-Time Integrator : DiscreteIntegrator  SampleTime=-1  ICPrevOutput=DiscIntNeverNeededParam  ICPrevScaledInput=DiscIntNeverNeededParam
  Scope1 : Scope  NumInputPorts=2
      settings: YMin=-5~-5  YMax=5~5  SaveName=ScopeData25
  SimLength : Constant  Value=SimLength
  ex_sfun_schedulefcn1 : S-Function  FunctionName=ex_sfun_schedulefcn  EnableBusSupport=off  mask(Legacy Function){SFunctionSpec=single y1 = schedule_fcn(double u1, double u2, single u3, single u4), ShowSpec=on}
      mask prompts: ShowSpec "Display function specification"
      mask help:
      | This block allows you to call the legacy functions specified by the following Legacy Code Tool definition:
      | def.SFunctionName = 'ex_sfun_schedulefcn';
      | def.OutputFcnSpec = 'single y1 = schedule_fcn(double u1, double u2, single u3, single u4)';
      | def.HeaderFiles = {'schedule_fcn.hpp'};
      | def.SourceFiles = {'schedule_fcn.cpp'};
      | def.Options.language = 'C++';
      mask Help: <p>This block was generated automatically by the Legacy Code Tool. For detailed help on this tool, call<a href="matlab:legacy_code('help')"> legacy_code('help')</a>.</p>
      mask Callback ShowSpec:
      | if strcmp(get_param(gcbh, 'ShowSpec'), 'on')
      |   set_param(gcbh, 'MaskDisplay', sprintf('fprintf(''%s'');', get_param(gcbh, 'SFunctionSpec')));
      | else
      |   set_param(gcbh, 'MaskDisplay', sprintf('fprintf(''%s'');', get_param(gcbh, 'FunctionName')));
      | end
      mask Display: fprintf('single y1 = schedule_fcn(double u1, double u2, single u3, single u4)');
  "fault_id " : Constant  Value=2  OutDataTypeStr=single
  one : Constant
  output : Outport  OutputWhenDisabled=reset  InitialOutput=[0]
  wires:
  one/1 -> Discrete-Time Integrator/1
  Discrete-Time Integrator/1 -> ex_sfun_schedulefcn1/2, Scope1/2
  ex_sfun_schedulefcn1/1 -> Scope1/1, output/1  "vcn_schedule"
  SimLength/1 -> ex_sfun_schedulefcn1/1
  "fault_id "/1 -> ex_sfun_schedulefcn1/3
  In1/1 -> ex_sfun_schedulefcn1/4

== system SensorFaultInj/FIM_Muster2/Parser Modul/schedule once per sample step /schedule_fcn id 3 ==
  In1 : Inport
  Discrete-Time Integrator : DiscreteIntegrator  SampleTime=-1  ICPrevOutput=DiscIntNeverNeededParam  ICPrevScaledInput=DiscIntNeverNeededParam
  Scope1 : Scope  NumInputPorts=2
      settings: YMin=-5~-5  YMax=5~5  SaveName=ScopeData25
  SimLength : Constant  Value=SimLength
  ex_sfun_schedulefcn1 : S-Function  FunctionName=ex_sfun_schedulefcn  EnableBusSupport=off  mask(Legacy Function){SFunctionSpec=single y1 = schedule_fcn(double u1, double u2, single u3, single u4), ShowSpec=on}
      mask prompts: ShowSpec "Display function specification"
      mask help:
      | This block allows you to call the legacy functions specified by the following Legacy Code Tool definition:
      | def.SFunctionName = 'ex_sfun_schedulefcn';
      | def.OutputFcnSpec = 'single y1 = schedule_fcn(double u1, double u2, single u3, single u4)';
      | def.HeaderFiles = {'schedule_fcn.hpp'};
      | def.SourceFiles = {'schedule_fcn.cpp'};
      | def.Options.language = 'C++';
      mask Help: <p>This block was generated automatically by the Legacy Code Tool. For detailed help on this tool, call<a href="matlab:legacy_code('help')"> legacy_code('help')</a>.</p>
      mask Callback ShowSpec:
      | if strcmp(get_param(gcbh, 'ShowSpec'), 'on')
      |   set_param(gcbh, 'MaskDisplay', sprintf('fprintf(''%s'');', get_param(gcbh, 'SFunctionSpec')));
      | else
      |   set_param(gcbh, 'MaskDisplay', sprintf('fprintf(''%s'');', get_param(gcbh, 'FunctionName')));
      | end
      mask Display: fprintf('single y1 = schedule_fcn(double u1, double u2, single u3, single u4)');
  "fault_id " : Constant  Value=3  OutDataTypeStr=single
  one : Constant
  output : Outport  OutputWhenDisabled=reset  InitialOutput=[0]
  wires:
  one/1 -> Discrete-Time Integrator/1
  Discrete-Time Integrator/1 -> ex_sfun_schedulefcn1/2, Scope1/2
  ex_sfun_schedulefcn1/1 -> Scope1/1, output/1  "tcn_schedule"
  SimLength/1 -> ex_sfun_schedulefcn1/1
  "fault_id "/1 -> ex_sfun_schedulefcn1/3
  In1/1 -> ex_sfun_schedulefcn1/4

== system SensorFaultInj/FIM_Muster2/Parser Modul/schedule once per sample step /schedule_fcn id 4 ==
  In1 : Inport
  Discrete-Time Integrator : DiscreteIntegrator  SampleTime=-1  ICPrevOutput=DiscIntNeverNeededParam  ICPrevScaledInput=DiscIntNeverNeededParam
  Scope1 : Scope  NumInputPorts=2
      settings: YMin=-5~-5  YMax=5~5  SaveName=ScopeData25
  SimLength : Constant  Value=SimLength
  ex_sfun_schedulefcn1 : S-Function  FunctionName=ex_sfun_schedulefcn  EnableBusSupport=off  mask(Legacy Function){SFunctionSpec=single y1 = schedule_fcn(double u1, double u2, single u3, single u4), ShowSpec=on}
      mask prompts: ShowSpec "Display function specification"
      mask help:
      | This block allows you to call the legacy functions specified by the following Legacy Code Tool definition:
      | def.SFunctionName = 'ex_sfun_schedulefcn';
      | def.OutputFcnSpec = 'single y1 = schedule_fcn(double u1, double u2, single u3, single u4)';
      | def.HeaderFiles = {'schedule_fcn.hpp'};
      | def.SourceFiles = {'schedule_fcn.cpp'};
      | def.Options.language = 'C++';
      mask Help: <p>This block was generated automatically by the Legacy Code Tool. For detailed help on this tool, call<a href="matlab:legacy_code('help')"> legacy_code('help')</a>.</p>
      mask Callback ShowSpec:
      | if strcmp(get_param(gcbh, 'ShowSpec'), 'on')
      |   set_param(gcbh, 'MaskDisplay', sprintf('fprintf(''%s'');', get_param(gcbh, 'SFunctionSpec')));
      | else
      |   set_param(gcbh, 'MaskDisplay', sprintf('fprintf(''%s'');', get_param(gcbh, 'FunctionName')));
      | end
      mask Display: fprintf('single y1 = schedule_fcn(double u1, double u2, single u3, single u4)');
  "fault_id " : Constant  Value=4  OutDataTypeStr=single
  one : Constant
  output : Outport  OutputWhenDisabled=reset  InitialOutput=[0]
  wires:
  one/1 -> Discrete-Time Integrator/1
  Discrete-Time Integrator/1 -> ex_sfun_schedulefcn1/2, Scope1/2
  ex_sfun_schedulefcn1/1 -> Scope1/1, output/1  "nco_schedule"
  SimLength/1 -> ex_sfun_schedulefcn1/1
  "fault_id "/1 -> ex_sfun_schedulefcn1/3
  In1/1 -> ex_sfun_schedulefcn1/4

== system SensorFaultInj/FIM_Muster2/Parser Modul/schedule once per sample step /schedule_fcn id 5 ==
  In1 : Inport
  Discrete-Time Integrator : DiscreteIntegrator  SampleTime=-1  ICPrevOutput=DiscIntNeverNeededParam  ICPrevScaledInput=DiscIntNeverNeededParam
  Scope1 : Scope  NumInputPorts=2
      settings: YMin=-5~-5  YMax=5~5  SaveName=ScopeData25
  SimLength : Constant  Value=SimLength
  ex_sfun_schedulefcn1 : S-Function  FunctionName=ex_sfun_schedulefcn  EnableBusSupport=off  mask(Legacy Function){SFunctionSpec=single y1 = schedule_fcn(double u1, double u2, single u3, single u4), ShowSpec=on}
      mask prompts: ShowSpec "Display function specification"
      mask help:
      | This block allows you to call the legacy functions specified by the following Legacy Code Tool definition:
      | def.SFunctionName = 'ex_sfun_schedulefcn';
      | def.OutputFcnSpec = 'single y1 = schedule_fcn(double u1, double u2, single u3, single u4)';
      | def.HeaderFiles = {'schedule_fcn.hpp'};
      | def.SourceFiles = {'schedule_fcn.cpp'};
      | def.Options.language = 'C++';
      mask Help: <p>This block was generated automatically by the Legacy Code Tool. For detailed help on this tool, call<a href="matlab:legacy_code('help')"> legacy_code('help')</a>.</p>
      mask Callback ShowSpec:
      | if strcmp(get_param(gcbh, 'ShowSpec'), 'on')
      |   set_param(gcbh, 'MaskDisplay', sprintf('fprintf(''%s'');', get_param(gcbh, 'SFunctionSpec')));
      | else
      |   set_param(gcbh, 'MaskDisplay', sprintf('fprintf(''%s'');', get_param(gcbh, 'FunctionName')));
      | end
      mask Display: fprintf('single y1 = schedule_fcn(double u1, double u2, single u3, single u4)');
  "fault_id " : Constant  Value=5  OutDataTypeStr=single
  one : Constant
  output : Outport  OutputWhenDisabled=reset  InitialOutput=[0]
  wires:
  one/1 -> Discrete-Time Integrator/1
  Discrete-Time Integrator/1 -> ex_sfun_schedulefcn1/2, Scope1/2
  ex_sfun_schedulefcn1/1 -> Scope1/1, output/1  "ncn_schedule"
  SimLength/1 -> ex_sfun_schedulefcn1/1
  "fault_id "/1 -> ex_sfun_schedulefcn1/3
  In1/1 -> ex_sfun_schedulefcn1/4
